simulink subsystem "DIG_IF"  (R2021b)
settings: Solver=VariableStepAuto  StartTime=0.0  StopTime=10.0  RelTol=1e-3
undefined symbols (not defined in the file or in its folder): combiner_attribs, dl_filter_attribs, splitter_attribs, ul_filter_attribs
settings Model: Creator=torha  LastModifiedBy=torha

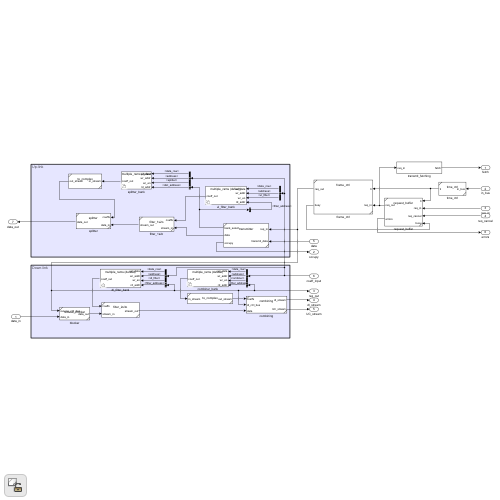
[thumbnail: Simulink's stored preview of the top-level diagram]
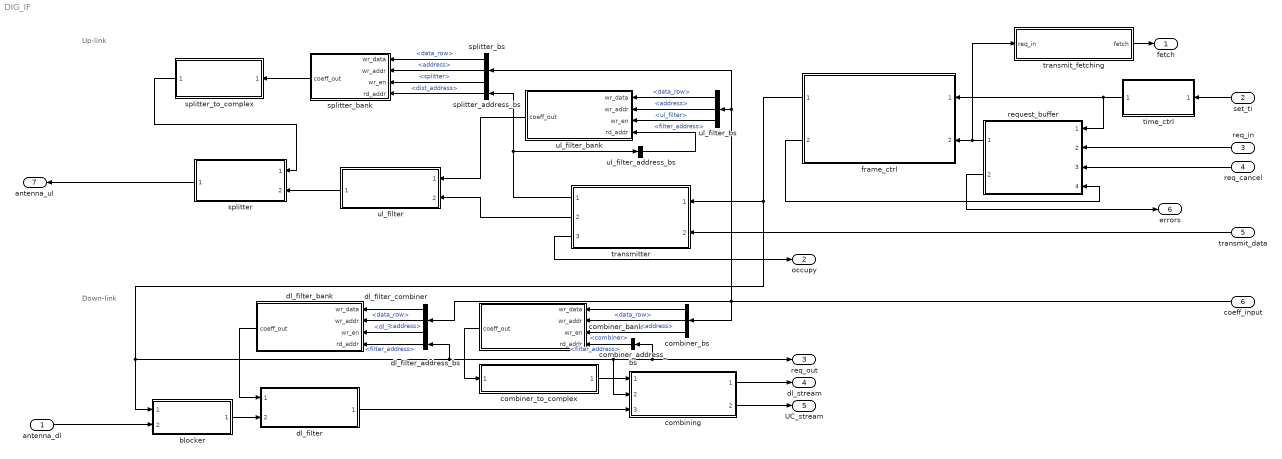
== system DIG_IF ==
  note: Up-link
  note: Down-link
  antenna_dl : Inport
  set_ti : Inport  Port=2
  req_in : Inport  Port=3
  req_cancel : Inport  Port=4
  transmit_data : Inport  Port=5
  coeff_input : Inport  Port=6
  blocker : Subsystem  ReferencedSubsystem=receive_blocker
  combiner_address_bs : BusSelector  OutputSignals=filter_address
  combiner_bank : Subsystem  Variant=on  mask{coeff=combiner_attribs}
      mask init:
      | load('constants.mat', 'coeff_ram_bitwidth');
      | last_ram_size = mod(coeff.coeff_bitwidth*coeff.coeff_num*(1+coeff.complex), coeff_ram_bitwidth);
      | if last_ram_size == 0
      |     last_ram_size = coeff_ram_bitwidth;
      | end
      | num_rams = ceil(coeff.coeff_bitwidth*coeff.coeff_num*(1+coeff.complex)/coeff_ram_bitwidth)-1;
  combiner_bs : BusSelector  OutputSignals=data_row,address,combiner
  combiner_to_complex : Subsystem  ReferencedSubsystem=to_complex
  combining : Subsystem  ReferencedSubsystem=combining
  dl_filter : Subsystem  ReferencedSubsystem=filter_2s3o
  dl_filter_address_bs : BusSelector  OutputSignals=filter_address
  dl_filter_bank : Subsystem  Variant=on  mask{coeff=dl_filter_attribs}
      mask init: same as DIG_IF/combiner_bank
  dl_filter_combiner : BusSelector  OutputSignals=data_row,address,dl_filter
  frame_ctrl : Subsystem  ReferencedSubsystem=frame_ctrl
  request_buffer : Subsystem  ReferencedSubsystem=request_buffer
  splitter : Subsystem  ReferencedSubsystem=splitter
  splitter_address_bs : BusSelector  OutputSignals=dist_address
  splitter_bank : Subsystem  Variant=on  mask{coeff=splitter_attribs}
      mask init: same as DIG_IF/combiner_bank
  splitter_bs : BusSelector  OutputSignals=data_row,address,splitter
  splitter_to_complex : Subsystem  ReferencedSubsystem=to_complex
  time_ctrl : Subsystem  ReferencedSubsystem=time_ctrl
  transmit_fetching : Subsystem
  transmitter : Subsystem  ReferencedSubsystem=transmitter
  ul_filter : Subsystem  ReferencedSubsystem=filter_2s3o
  ul_filter_address_bs : BusSelector  OutputSignals=filter_address
  ul_filter_bank : Subsystem  Variant=on  mask{coeff=ul_filter_attribs}
      mask init: same as DIG_IF/combiner_bank
  ul_filter_bs : BusSelector  OutputSignals=data_row,address,ul_filter
  fetch : Outport
  occupy : Outport  Port=2
  req_out : Outport  Port=3
  dl_stream : Outport  Port=4
  UC_stream : Outport  Port=5
  errors : Outport  Port=6
  antenna_ul : Outport  Port=7
  wires:
  frame_ctrl/2 -> request_buffer/4
  combiner_bs/1 -> combiner_bank/1(wr_data)  "<data_row>"
  transmitter/1 -> splitter_address_bs/1, ul_filter_address_bs/1
  dl_filter/1 -> combining/3
  dl_filter_address_bs/1 -> dl_filter_bank/4(rd_addr)  "<filter_address>"
  dl_filter_bank/1(coeff_out) -> dl_filter/1
  combiner_bs/3 -> combiner_bank/3(wr_en)  "<combiner>"
  dl_filter_combiner/3 -> dl_filter_bank/3(wr_en)  "<dl_filter>"
  request_buffer/1 -> transmit_fetching/1(req_in), frame_ctrl/2
  frame_ctrl/1 -> blocker/1, dl_filter_address_bs/1, combining/2, combiner_address_bs/1, req_out/1, transmitter/1
  ul_filter_bs/3 -> ul_filter_bank/3(wr_en)  "<ul_filter>"
  time_ctrl/1 -> frame_ctrl/1, request_buffer/1
  ul_filter_bs/1 -> ul_filter_bank/1(wr_data)  "<data_row>"
  transmit_data/1 -> transmitter/2
  combiner_address_bs/1 -> combiner_bank/4(rd_addr)  "<filter_address>"
  splitter_bank/1(coeff_out) -> splitter_to_complex/1
  blocker/1 -> dl_filter/2
  combining/1 -> dl_stream/1
  splitter_bs/1 -> splitter_bank/1(wr_data)  "<data_row>"
  antenna_dl/1 -> blocker/2
  splitter_to_complex/1 -> splitter/1
  dl_filter_combiner/1 -> dl_filter_bank/1(wr_data)  "<data_row>"
  splitter_bs/3 -> splitter_bank/3(wr_en)  "<splitter>"
  coeff_input/1 -> combiner_bs/1, dl_filter_combiner/1, splitter_bs/1, ul_filter_bs/1
  dl_filter_combiner/2 -> dl_filter_bank/2(wr_addr)  "<address>"
  req_cancel/1 -> request_buffer/3
  ul_filter_bank/1(coeff_out) -> ul_filter/1
  splitter_address_bs/1 -> splitter_bank/4(rd_addr)  "<dist_address>"
  combining/2 -> UC_stream/1
  splitter_bs/2 -> splitter_bank/2(wr_addr)  "<address>"
  ul_filter_address_bs/1 -> ul_filter_bank/4(rd_addr)  "<filter_address>"
  transmit_fetching/1(fetch) -> fetch/1
  combiner_bank/1(coeff_out) -> combiner_to_complex/1
  combiner_bs/2 -> combiner_bank/2(wr_addr)  "<address>"
  combiner_to_complex/1 -> combining/1
  splitter/1 -> antenna_ul/1
  transmitter/2 -> ul_filter/2
  ul_filter_bs/2 -> ul_filter_bank/2(wr_addr)  "<address>"
  ul_filter/1 -> splitter/2
  set_ti/1 -> time_ctrl/1
  transmitter/3 -> occupy/1
  request_buffer/2 -> errors/1
  req_in/1 -> request_buffer/2

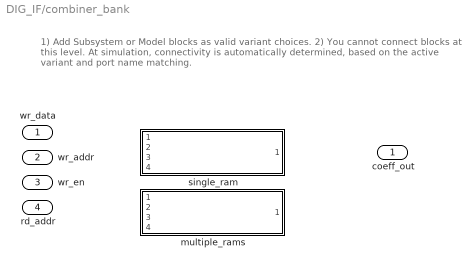
== system DIG_IF/combiner_bank ==
  note: 1) Add Subsystem or Model blocks as valid variant choices.
      | 2) You cannot connect blocks at this level. At simulation, connectivity is automatically
      | determined, based on the active variant and port name matching.
  wr_data : Inport
  wr_addr : Inport  Port=2
  wr_en : Inport  Port=3
  rd_addr : Inport  Port=4
  multiple_rams : Subsystem  VariantControl=(default)  ReferencedSubsystem=coeff_bank_multiple_rams
  single_ram : Subsystem  VariantControl=num_rams==0  ReferencedSubsystem=coeff_bank_single_ram
  coeff_out : Outport

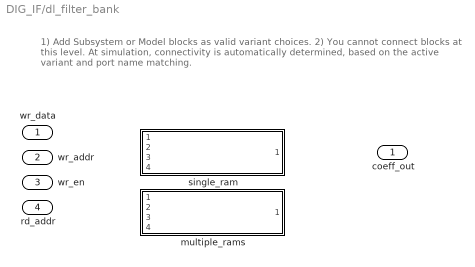
== system DIG_IF/dl_filter_bank ==
  note: 1) Add Subsystem or Model blocks as valid variant choices.
      | 2) You cannot connect blocks at this level. At simulation, connectivity is automatically
      | determined, based on the active variant and port name matching.
  wr_data : Inport
  wr_addr : Inport  Port=2
  wr_en : Inport  Port=3
  rd_addr : Inport  Port=4
  multiple_rams : Subsystem  VariantControl=(default)  ReferencedSubsystem=coeff_bank_multiple_rams
  single_ram : Subsystem  VariantControl=num_rams==0  ReferencedSubsystem=coeff_bank_single_ram
  coeff_out : Outport

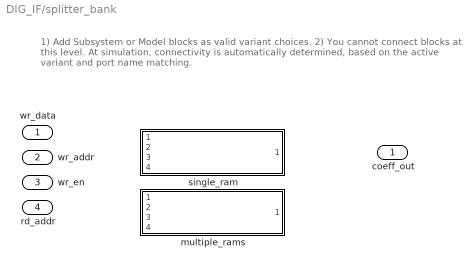
== system DIG_IF/splitter_bank ==
  note: 1) Add Subsystem or Model blocks as valid variant choices.
      | 2) You cannot connect blocks at this level. At simulation, connectivity is automatically
      | determined, based on the active variant and port name matching.
  wr_data : Inport
  wr_addr : Inport  Port=2
  wr_en : Inport  Port=3
  rd_addr : Inport  Port=4
  multiple_rams : Subsystem  VariantControl=(default)  ReferencedSubsystem=coeff_bank_multiple_rams
  single_ram : Subsystem  VariantControl=num_rams==0  ReferencedSubsystem=coeff_bank_single_ram
  coeff_out : Outport

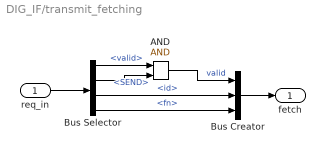
== system DIG_IF/transmit_fetching ==
  req_in : Inport
  AND : Logic  IconShape=distinctive  AllPortsSameDT=off  OutDataTypeStr=boolean
  Bus Creator : BusCreator  Inputs=3
  Bus Selector : BusSelector  OutputSignals=valid,req.SEND,id,req.fn
  fetch : Outport
  wires:
  Bus Selector/4 -> Bus Creator/3  "<fn>"
  Bus Creator/1 -> fetch/1
  Bus Selector/3 -> Bus Creator/2  "<id>"
  AND/1 -> Bus Creator/1  "valid"
  Bus Selector/1 -> AND/1  "<valid>"
  Bus Selector/2 -> AND/2  "<SEND>"
  req_in/1 -> Bus Selector/1

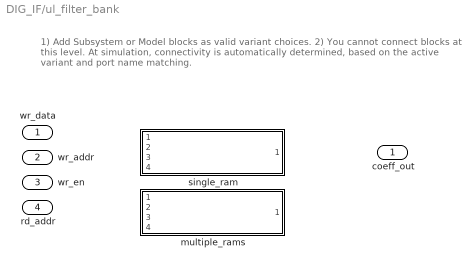
== system DIG_IF/ul_filter_bank ==
  note: 1) Add Subsystem or Model blocks as valid variant choices.
      | 2) You cannot connect blocks at this level. At simulation, connectivity is automatically
      | determined, based on the active variant and port name matching.
  wr_data : Inport
  wr_addr : Inport  Port=2
  wr_en : Inport  Port=3
  rd_addr : Inport  Port=4
  multiple_rams : Subsystem  VariantControl=(default)  ReferencedSubsystem=coeff_bank_multiple_rams
  single_ram : Subsystem  VariantControl=num_rams==0  ReferencedSubsystem=coeff_bank_single_ram
  coeff_out : Outport
